simulink model "mpc_ydx_control"  (R2022b)
settings: Solver=VariableStepAuto  StartTime=0.0  StopTime=50  RelTol=1e-3
values from neighbouring files (symbols this model uses):
  cx = 0:0.1:120    [mpcdlx_ref.m]
libraries: Solver_SF x1, simulink x1
settings Model: Creator=admin  LastModifiedBy=admin

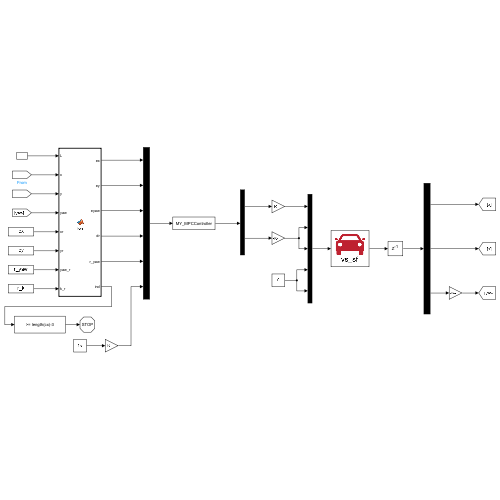
[thumbnail: Simulink's stored preview of the top-level diagram]
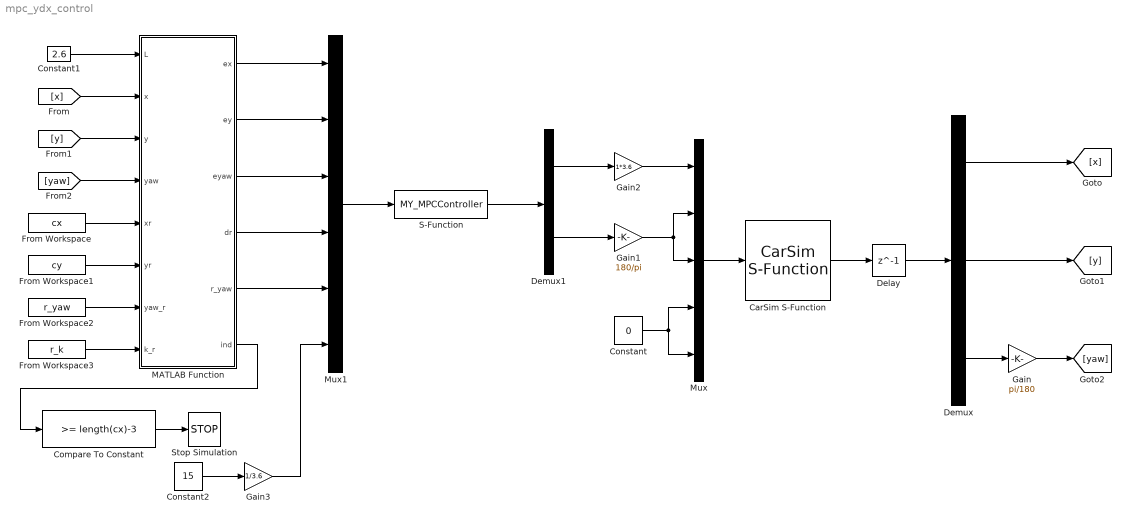
== system mpc_ydx_control ==
  CarSim S-Function : Solver_SF/CarSim S-Function  Priority=1  SIMFILE=simfile.sim  Run_RTs=off  vs_state_ind=Run  StopMode_ind=Vehicle Model
  Compare To Constant : simulink/Logic and Bit Operations/Compare To Constant  relop=>=  const=length(cx)-3  OutDataTypeStr=boolean
  Constant : Constant  Value=0
  Constant1 : Constant  Value=2.6
  Constant2 : Constant  Value=15
  Delay : Delay  DelayLength=1
  Demux : Demux  Outputs=3
  Demux1 : Demux  Outputs=2
  From Workspace : FromWorkspace  VariableName=cx
  From Workspace1 : FromWorkspace  VariableName=cy
  From Workspace2 : FromWorkspace  VariableName=r_yaw
  From Workspace3 : FromWorkspace  VariableName=r_k
  Gain : Gain  Gain=pi/180
  Gain1 : Gain  Gain=180/pi
  Gain2 : Gain  Gain=1*3.6
  Gain3 : Gain  Gain=1/3.6
  MATLAB Function : MATLAB Function  TreatAsAtomicUnit=on
  Mux : Mux  Inputs=5
  Mux1 : Mux  Inputs=6
  S-Function : S-Function  FunctionName=MY_MPCController  SFunctionDeploymentMode=off  EnableBusSupport=off
  Stop Simulation : Stop
  wires:
  CarSim S-Function/1 -> Delay/1
  Delay/1 -> Demux/1
  Demux/1 -> [x]
  Demux/2 -> [y]
  Gain/1 -> [yaw]
  Demux/3 -> Gain/1
  Mux/1 -> CarSim S-Function/1
  Constant/1 -> Mux/5, Mux/4
  Gain1/1 -> Mux/2, Mux/3
  Gain2/1 -> Mux/1
  Constant1/1 -> MATLAB Function/1(L)
  [x] -> MATLAB Function/2(x)
  [y] -> MATLAB Function/3(y)
  [yaw] -> MATLAB Function/4(yaw)
  From Workspace/1 -> MATLAB Function/5(xr)
  From Workspace1/1 -> MATLAB Function/6(yr)
  From Workspace2/1 -> MATLAB Function/7(yaw_r)
  From Workspace3/1 -> MATLAB Function/8(k_r)
  MATLAB Function/1(ex) -> Mux1/1
  MATLAB Function/2(ey) -> Mux1/2
  MATLAB Function/3(eyaw) -> Mux1/3
  MATLAB Function/4(dr) -> Mux1/4
  MATLAB Function/5(r_yaw) -> Mux1/5
  MATLAB Function/6(ind) -> Compare To Constant/1
  Constant2/1 -> Gain3/1
  Gain3/1 -> Mux1/6
  Compare To Constant/1 -> Stop Simulation/1
  Mux1/1 -> S-Function/1
  Demux1/1 -> Gain2/1
  Demux1/2 -> Gain1/1
  S-Function/1 -> Demux1/1

== matlab function mpc_ydx_control/MATLAB Function ==
  data: L input; ex output; x input; y input; yaw input; xr input; yr input; yaw_r input; k_r input; ey output; eyaw output; dr output; r_yaw output; ind output
function [ex,ey,eyaw,dr,r_yaw,ind] = fcn(L,x,y,yaw,xr,yr,yaw_r,k_r)
%1.寻找匹配点（车辆离期望路径最近的点）   
    n=length(xr);
    d_min=(x-xr(1))^2+(y-yr(1))^2;
    min=1;
    for i=1:n
        d=(x-xr(i))^2+(y-yr(i))^2;
        if d<d_min
            d_min=d;
            min=i;
        end
    end
    ind=min;

%2.计算3个误差状态[ex,ey,eyaw]
    ex=x-xr(ind);
    ey=y-yr(ind);

    eyaw=yaw-yaw_r(ind);

%3.计算计算参考前轮转角dr
    dr=atan(L*k_r(ind));

%4.参考航向角也输出  
    r_yaw=yaw_r(ind);

end
